simulink model "validacaoDCDC"  (R2018a)
settings: Solver=ode23t  StartTime=0.0  StopTime=0.1  MaxStep=1e-4  RelTol=1e-3  EnableMultiTasking=on
PreLoadFcn:
  | SRated = 150e3; % W
  | VRated = 440; % V
  | FRated = 60; % Hz
  | 
  | QNominal = sin(acos(0.8))*SRated;
  | QPerPhase = QNominal / 3;
  | 
  | IPerPhase = QPerPhase/VRated;
  | Xc = VRated/IPerPhase;
  | reactiveCompensationCapacitance = 1/(2*pi*FRated*Xc);
  | 
  | clear( 'QNominal', 'QPerPhase', 'IPerPhase', 'Xc' );
libraries: powerlib x7, powerlib_meascontrol x1
Description:
  | Three-Phase Asynchronous Wind Turbine Generator
  | 
  | This example shows an induction machine used as a wind turbine generator.
  | The Simple Turbine block converts wind speed to turbine output power by a
  | simple output power versus wind speed characteristic.
  | 
  | When the wind speed is below the cut-in speed or above the cut-out speed,
  | the machine generates zero real power. The machine always consumes
  | reactive power. The Reactive Compensation block offsets the machine's
  | reactive power requirement.
  | 
  | The local load consumes 75kW. The infeed from the power grid meets any
  | wind turbine generation shortfall. When the generator produces more than
  | 75kW, excess power is exported to the grid.
  | 
  | Copyright 2014-2017 The MathWorks, Inc.
settings Model: Creator=The MathWorks, Inc.  LastModifiedBy=VMORAIS
settings DataIOCC: LimitDataPoints=on  SaveFormat=Array  SaveOutput=off  SignalLogging=off  DSMLogging=off  SaveTime=off
settings OptimizationCC: LifeSpan=inf
settings DebuggingCC: UnderspecifiedInitializationDetection=Classic  MergeDetectMultiDrivingBlocksExec=none  SFUnexpectedBacktrackingDiag=warning  SFNoUnconditionalDefaultTransitionDiag=warning  SFExecutionAtInitializationDiag=none
settings HardwareCC: ProdBitPerPointer=32  ProdBitPerSizeT=32  ProdBitPerPtrDiffT=32  ProdLargestAtomicFloat=None  ProdIntDivRoundTo=Undefined  ProdEndianess=Unspecified  ProdWordSize=32  ProdHWDeviceType=32-bit Generic
settings ModelReferenceCC: PropagateSignalLabelsOutOfModel=off
settings CodeAppCC: StateflowObjectComments=on
settings GRTTargetCC: TargetLangStandard=C89/C90 (ANSI)  GeneratePreprocessorConditionals=Disable all
settings ConfigComp: CovMetricSettings=dw  CovHtmlReporting=on  CovSaveCumulativeToWorkspaceVar=on  CovSaveSingleToWorkspaceVar=on  CovExternalEMLEnable=off  CovSFcnEnable=off
settings SimscapeCC: SimscapeLogSimulationStatistics=on  SimscapeLogOpenViewer=on  SimscapeLogLimitData=off

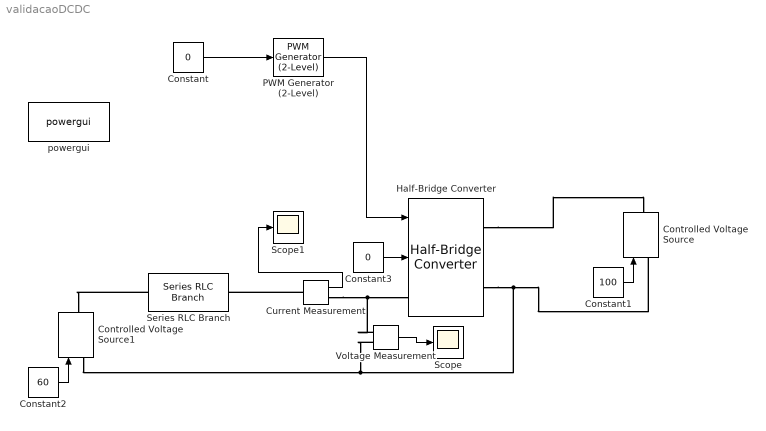
== system validacaoDCDC ==
  Constant : Constant  Value=0
  Constant1 : Constant  Value=100
  Constant2 : Constant  Value=60
  Constant3 : Constant  Value=0
  Controlled Voltage Source : powerlib/Electrical Sources/Controlled Voltage Source  Initialize=on  Source_Type=DC  Amplitude=100  Phase=0  Frequency=0  Measurements=None
  Controlled Voltage Source1 : powerlib/Electrical Sources/Controlled Voltage Source  Initialize=on  Source_Type=DC  Amplitude=100  Phase=0  Frequency=0  Measurements=None
  Current Measurement : powerlib/Measurements/Current Measurement  PhasorSimulation=off  OutputType=Complex  PSBequivalent=0
  Half-Bridge Converter : powerlib/Power Electronics/Half-Bridge Converter  ModelType=Switching devices  Ron=1e-3  Rs=1e6  Cs=inf  Vforward=[0,0]  Ron_Diode=1e-3  Rs_Diode=1e6  Cs_Diode=inf  Vf_Diode=1e-3  Rs_CurrentSource=inf
      settings: SourceProductName=Simscape Power Systems  SourceProductBaseCode=PS
  PWM Generator (2-Level) : powerlib_meascontrol/Pulse & Signal Generators/PWM Generator (2-Level)  ModulatorType=Single-phase half-bridge (2 pulses)  ModulatorMode=Unsynchronized  Fc=10e3  Pc=90  nF=27  MinMax="[ -1  1 ]"  SamplingTechnique=Natural  ModulatingSignals=off  m=0.8  Freq=60  Phase=0  Ts=0  ShowCarrierOutport=off
      settings: SourceProductName=Simscape Power Systems
  Scope : Scope
  Scope1 : Scope
  Series RLC Branch : powerlib/Elements/Series RLC Branch  LConnTagsString=__new0  RConnTagsString=__new0  BranchType=RL  Resistance=0.1  Inductance=1e-3  SetiL0=off  InitialCurrent=0  Capacitance=1e-6  Setx0=off  InitialVoltage=0  Measurements=None
  Voltage Measurement : powerlib/Measurements/Voltage Measurement  PhasorSimulation=off  OutputType=Complex  PSBequivalent=0
  powergui : powerlib/powergui  Priority=1  SimulationMode=Continuous  SampleTime=50e-6  frequency=60  Iterations=50  frequencyindice=0  Pbase=100e6  ErrMax=1e-4  UnitsV=kV  UnitsW=MW  buscounter=0  FunctionMessages=off  echomessages=off  EnableUseOfTLC=off  CurrentSourceSwitches=off  DisableSnubberDevices=off  DisableRonSwitches=off  DisableVfSwitches=off  DisplayEquations=off  SolverType=Tustin/Backward Euler (TBE)  Interpol=off  ExternalGateDelay=off  methode=off  Ts=100  x0status=blocks  SPID=on  SwTol=0  HookPort=off  RestoreLinks=warning  ResistiveCurrentMeasurement=off  Frange=[0:2:500]  Ylog=off  Xlog=on  ShowGrid=off  save=off  variable=ZData  structure=0  ZoomFFT=off  StartTime=0.0  cycles=1  DisplayStyle=1  fundamental=60  FreqAxis=off  MaxFrequency=1000  frequencyindicesteady=1  RmsSteady=1  display=off
  wires:
  Constant/1 -> PWM Generator (2-Level)/1
  Constant1/1 -> Controlled Voltage Source/1
  Constant2/1 -> Controlled Voltage Source1/1
  Current Measurement/1 -> Scope1/1
  Constant3/1 -> Half-Bridge Converter/2
  PWM Generator (2-Level)/1 -> Half-Bridge Converter/1
  Voltage Measurement/1 -> Scope/1
  connections:
  Half-Bridge Converter/RConn1 -- Controlled Voltage Source/RConn1
  Half-Bridge Converter/RConn2 -- Voltage Measurement/LConn2 -- Controlled Voltage Source1/LConn1 -- Controlled Voltage Source/LConn1
  Current Measurement/LConn1 -- Series RLC Branch/RConn1
  Current Measurement/RConn1 -- Voltage Measurement/LConn1 -- Half-Bridge Converter/LConn1
  Series RLC Branch/LConn1 -- Controlled Voltage Source1/RConn1
